simulink model "Roadsense_LocalPlanner"  (R2025b)
settings: Solver=FixedStepDiscrete  StartTime=0.0  StopTime=1.0  FixedStep=RsTsBase  RelTol=1e-3
undefined symbols (not defined in the file or in its folder): RsGridCols, RsGridRows, RsMaxPlanPoints, RsMaxPredictionModes, RsMaxReferencePoints, RsMaxTracks, RsPredictionSteps, RsTsPlanning
settings Model: DataDictionary=Roadsense_Data.sldd  Creator=ragur  LastModifiedBy=ragur

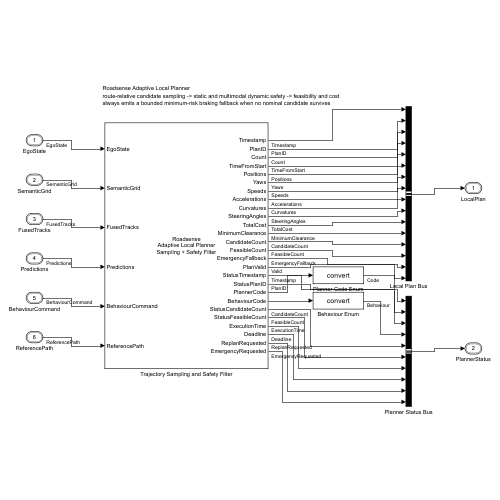
[thumbnail: Simulink's stored preview of the top-level diagram]
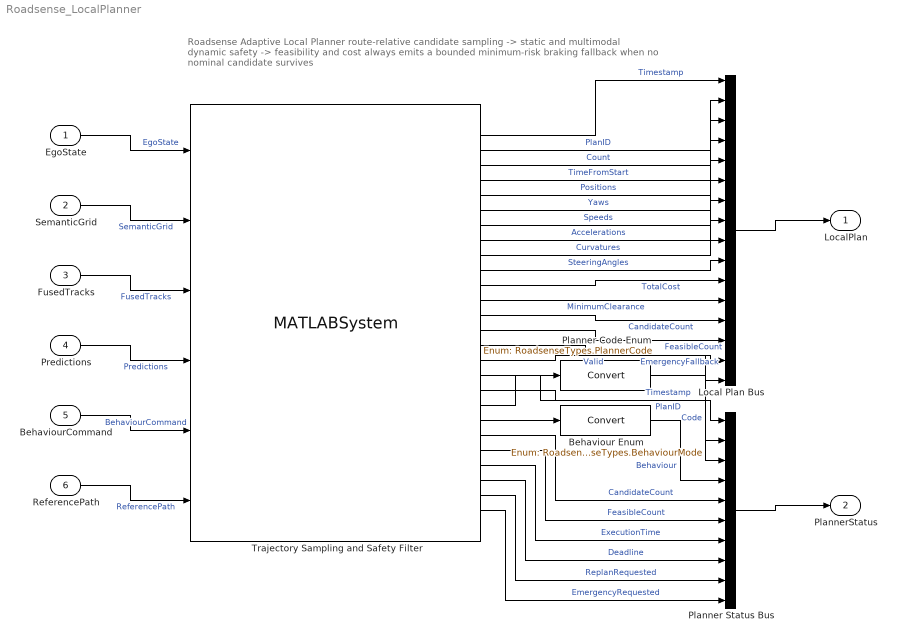
== system Roadsense_LocalPlanner ==
  note: Roadsense Adaptive Local Planner
      | route-relative candidate sampling -> static and multimodal dynamic safety -> feasibility and cost
      | always emits a bounded minimum-risk braking fallback when no nominal candidate survives
  EgoState : Inport  OutDataTypeStr=Bus: RsEgoStateBus  PortDimensions=1  SampleTime=RsTsPlanning
  SemanticGrid : Inport  Port=2  OutDataTypeStr=Bus: RsSemanticGridBus  PortDimensions=1  SampleTime=RsTsPlanning
  FusedTracks : Inport  Port=3  OutDataTypeStr=Bus: RsFusedTrackListBus  PortDimensions=1  SampleTime=RsTsPlanning
  Predictions : Inport  Port=4  OutDataTypeStr=Bus: RsMotionPredictionListBus  PortDimensions=1  SampleTime=RsTsPlanning
  BehaviourCommand : Inport  Port=5  OutDataTypeStr=Bus: RsBehaviourCommandBus  PortDimensions=1  SampleTime=RsTsPlanning
  ReferencePath : Inport  Port=6  OutDataTypeStr=Bus: RsReferencePathBus  PortDimensions=1  SampleTime=RsTsPlanning
  Behaviour Enum : DataTypeConversion  OutDataTypeStr=Enum: RoadsenseTypes.BehaviourMode  SaturateOnIntegerOverflow=off  RndMeth=Floor
  Local Plan Bus : BusCreator  Inputs=16  OutDataTypeStr=Bus: RsLocalPlanBus
  Planner Code Enum : DataTypeConversion  OutDataTypeStr=Enum: RoadsenseTypes.PlannerCode  SaturateOnIntegerOverflow=off  RndMeth=Floor
  Planner Status Bus : BusCreator  Inputs=10  OutDataTypeStr=Bus: RsPlannerStatusBus
  Trajectory Sampling and Safety Filter : MATLABSystem  System=RoadsenseLocalPlannerSystem  MaxPlanPoints=double(RsMaxPlanPoints)  MaxReferencePoints=double(RsMaxReferencePoints)  MaxTracks=double(RsMaxTracks)  MaxModes=double(RsMaxPredictionModes)  PredictionSteps=double(RsPredictionSteps)  GridRows=double(RsGridRows)  GridCols=double(RsGridCols)  PlanStep=RsPlanStep  PlanHorizon=RsPlanHorizon  LateralTransitionDistance=RsPlannerLateralTransitionDistance  LateralOffsets=RsPlannerLateralOffsets  SpeedScales=RsPlannerSpeedScales  Wheelbase=RsPlannerWheelbase  VehicleLength=RsPlannerVehicleLength  VehicleWidth=RsPlannerVehicleWidth  MaximumCurvature=RsPlannerMaximumCurvature  MaximumJerk=RsPlannerMaximumJerk  HardOccupancy=RsPlannerHardOccupancy  CollisionProbability=RsPlannerCollisionProbability  PredictionSigma=RsPlannerPredictionSigma  MaximumLongitudinalInflation=RsPlannerMaximumLongitudinalInflation  MaximumLateralInflation=RsPlannerMaximumLateralInflation  LateralClearanceRatio=RsPlannerLateralClearanceRatio  MaximumLateralClearance=RsPlannerMaximumLateralClearance  Deadline=RsPlannerDeadline  SimulateUsing=Code generation
      mask Type: RoadsenseLocalPlannerSystem
  LocalPlan : Outport  OutDataTypeStr=Bus: RsLocalPlanBus
  PlannerStatus : Outport  Port=2  OutDataTypeStr=Bus: RsPlannerStatusBus
  wires:
  EgoState/1 -> Trajectory Sampling and Safety Filter/1  "EgoState"
  SemanticGrid/1 -> Trajectory Sampling and Safety Filter/2  "SemanticGrid"
  FusedTracks/1 -> Trajectory Sampling and Safety Filter/3  "FusedTracks"
  Predictions/1 -> Trajectory Sampling and Safety Filter/4  "Predictions"
  BehaviourCommand/1 -> Trajectory Sampling and Safety Filter/5  "BehaviourCommand"
  ReferencePath/1 -> Trajectory Sampling and Safety Filter/6  "ReferencePath"
  Trajectory Sampling and Safety Filter/19 -> Planner Code Enum/1
  Trajectory Sampling and Safety Filter/20 -> Behaviour Enum/1
  Trajectory Sampling and Safety Filter/1 -> Local Plan Bus/1  "Timestamp"
  Trajectory Sampling and Safety Filter/2 -> Local Plan Bus/2  "PlanID"
  Trajectory Sampling and Safety Filter/3 -> Local Plan Bus/3  "Count"
  Trajectory Sampling and Safety Filter/4 -> Local Plan Bus/4  "TimeFromStart"
  Trajectory Sampling and Safety Filter/5 -> Local Plan Bus/5  "Positions"
  Trajectory Sampling and Safety Filter/6 -> Local Plan Bus/6  "Yaws"
  Trajectory Sampling and Safety Filter/7 -> Local Plan Bus/7  "Speeds"
  Trajectory Sampling and Safety Filter/8 -> Local Plan Bus/8  "Accelerations"
  Trajectory Sampling and Safety Filter/9 -> Local Plan Bus/9  "Curvatures"
  Trajectory Sampling and Safety Filter/10 -> Local Plan Bus/10  "SteeringAngles"
  Trajectory Sampling and Safety Filter/11 -> Local Plan Bus/11  "TotalCost"
  Trajectory Sampling and Safety Filter/12 -> Local Plan Bus/12  "MinimumClearance"
  Trajectory Sampling and Safety Filter/13 -> Local Plan Bus/13  "CandidateCount"
  Trajectory Sampling and Safety Filter/14 -> Local Plan Bus/14  "FeasibleCount"
  Trajectory Sampling and Safety Filter/15 -> Local Plan Bus/15  "EmergencyFallback"
  Trajectory Sampling and Safety Filter/16 -> Local Plan Bus/16  "Valid"
  Trajectory Sampling and Safety Filter/17 -> Planner Status Bus/1  "Timestamp"
  Trajectory Sampling and Safety Filter/18 -> Planner Status Bus/2  "PlanID"
  Planner Code Enum/1 -> Planner Status Bus/3  "Code"
  Behaviour Enum/1 -> Planner Status Bus/4  "Behaviour"
  Trajectory Sampling and Safety Filter/21 -> Planner Status Bus/5  "CandidateCount"
  Trajectory Sampling and Safety Filter/22 -> Planner Status Bus/6  "FeasibleCount"
  Trajectory Sampling and Safety Filter/23 -> Planner Status Bus/7  "ExecutionTime"
  Trajectory Sampling and Safety Filter/24 -> Planner Status Bus/8  "Deadline"
  Trajectory Sampling and Safety Filter/25 -> Planner Status Bus/9  "ReplanRequested"
  Trajectory Sampling and Safety Filter/26 -> Planner Status Bus/10  "EmergencyRequested"
  Local Plan Bus/1 -> LocalPlan/1
  Planner Status Bus/1 -> PlannerStatus/1
